simulink model "motor_plant"  (R2023b)
settings: Solver=VariableStepAuto  StartTime=0.0  StopTime=10.0  RelTol=1e-3
InitFcn:
  | %%%%%%%%%%%%%%%%%%%%%%%%%%%%%%%%%%%%%%%%%%%%%%%%%
  | %motor parameters
  | %we dont know these yet
  | J = 1e-6; %intertia [kg * m^2]
  | Bm = 1e-6; %kinetic friction [N * m * s]
  | 
  | %from motor datasheet
  | Km = 0.011; %motor constant (back emf constant = torque constant)
  | Rw = 1.17; %motor electric resistance in ohms
  | Lw = 0.58E-3; %motor inductance in ohms
settings Model: Creator=you29  LastModifiedBy=you29

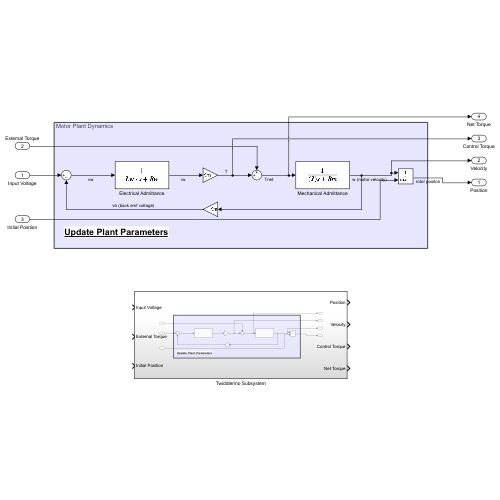
[thumbnail: Simulink's stored preview of the top-level diagram]
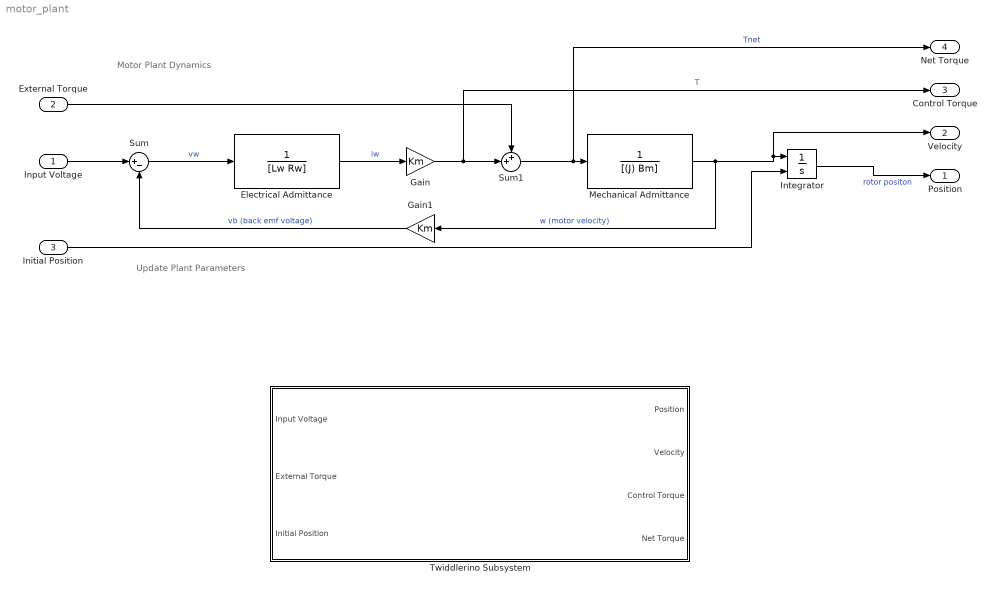
== system motor_plant ==
  note: Update Plant Parameters
  note: Motor Plant Dynamics
  Input Voltage : Inport
  External Torque : Inport  Port=2
  Initial Position : Inport  Port=3
  Electrical Admittance : TransferFcn  Denominator=[Lw Rw]
  Gain : Gain  Gain=Km
  Gain1 : Gain  Gain=Km
  Integrator : Integrator  InitialConditionSource=external
  Mechanical Admittance : TransferFcn  Denominator=[(J) Bm]
  Sum : Sum  Inputs=|+-
  Sum1 : Sum  Inputs=++|
  Twiddlerino Subsystem : Subsystem
  Position : Outport
  Velocity : Outport  Port=2
  Control Torque : Outport  Port=3
  Net Torque : Outport  Port=4
  wires:
  Input Voltage/1 -> Sum/1
  Sum/1 -> Electrical Admittance/1  "vw"
  Electrical Admittance/1 -> Gain/1  "iw"
  Gain/1 -> Control Torque/1, Sum1/2  "T"
  External Torque/1 -> Sum1/1
  Sum1/1 -> Net Torque/1, Mechanical Admittance/1  "Tnet"
  Mechanical Admittance/1 -> Velocity/1, Integrator/1, Gain1/1  "w (motor velocity)"
  Gain1/1 -> Sum/2  "vb (back emf voltage)"
  Integrator/1 -> Position/1  "rotor positon"
  Initial Position/1 -> Integrator/2

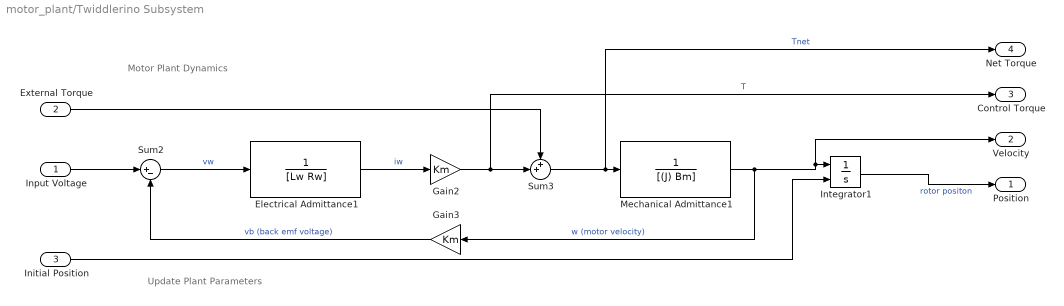
== system motor_plant/Twiddlerino Subsystem ==
  note: Update Plant Parameters
  note: Motor Plant Dynamics
  Input Voltage : Inport
  External Torque : Inport  Port=2
  Initial Position : Inport  Port=3
  Electrical Admittance1 : TransferFcn  Denominator=[Lw Rw]
  Gain2 : Gain  Gain=Km
  Gain3 : Gain  Gain=Km
  Integrator1 : Integrator  InitialConditionSource=external
  Mechanical Admittance1 : TransferFcn  Denominator=[(J) Bm]
  Sum2 : Sum  Inputs=|+-
  Sum3 : Sum  Inputs=++|
  Position : Outport
  Velocity : Outport  Port=2
  Control Torque : Outport  Port=3
  Net Torque : Outport  Port=4
  wires:
  Initial Position/1 -> Integrator1/2
  Sum3/1 -> Net Torque/1, Mechanical Admittance1/1  "Tnet"
  Electrical Admittance1/1 -> Gain2/1  "iw"
  External Torque/1 -> Sum3/1
  Mechanical Admittance1/1 -> Velocity/1, Integrator1/1, Gain3/1  "w (motor velocity)"
  Gain3/1 -> Sum2/2  "vb (back emf voltage)"
  Sum2/1 -> Electrical Admittance1/1  "vw"
  Input Voltage/1 -> Sum2/1
  Integrator1/1 -> Position/1  "rotor positon"
  Gain2/1 -> Control Torque/1, Sum3/2  "T"
